simulink model "flux_control_example"  (Simulink 6.3)
settings: Solver=ode3  SolverMode=SingleTasking  StartTime=0.0  StopTime=2  FixedStep=0.02  MaxStep=0.1  MinStep=1e-2  RelTol=1e-2
libraries: simulink x21
settings Model: Creator=JA132999  LastModifiedBy=JA132999  ExtModeAutoUpdateStatusClock=off  BufferReuse=off
settings SolverCC: InitialStep=1e-2
settings MATStruct: SampleTime=0.01  Offset=0  Priority=[1.0]
settings OptimizationCC: BlockReduction=off  BooleanDataType=off  ConditionallyExecuteInputs=off  OptimizeBlockIOStorage=off  BufferReuse=off  ExpressionFolding=off  LocalBlockOutputs=off

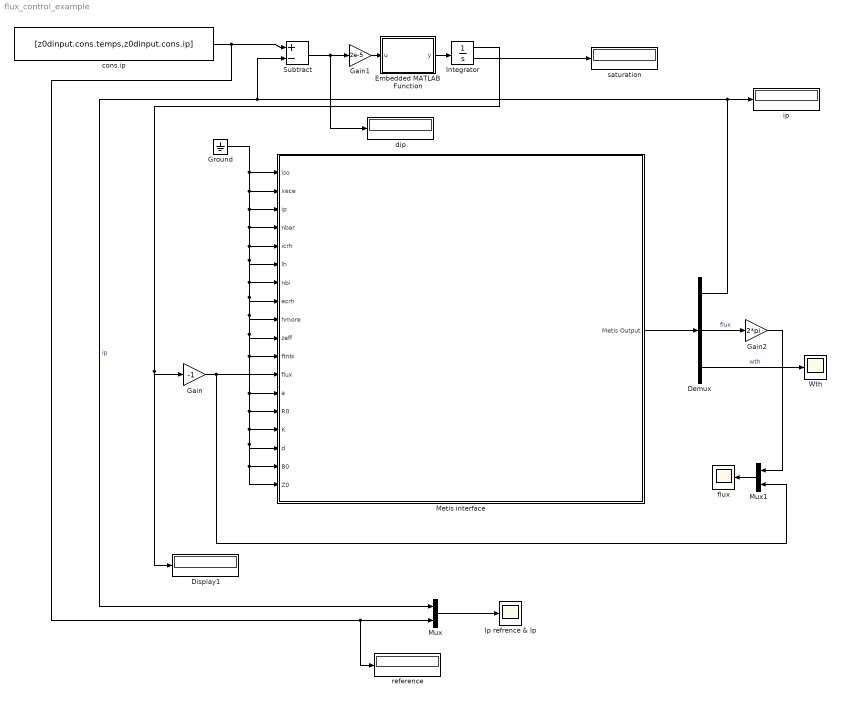
== system flux_control_example ==
  Demux : Demux  Outputs=3
  Display1 : Display
  Embedded MATLAB Function : Stateflow chart
  Gain : Gain  Gain=-1
  Gain1 : Gain  Gain=2e-5
  Gain2 : Gain  Gain=2*pi
  Ground : Ground
  Integrator : Integrator  ShowSaturationPort=on  ZeroCross=off
  Ip refrence & Ip : Scope
      settings: YMin=0  YMax=800000  SaveName=ScopeData3
  Metis interface : Subsystem  AncestorBlock=library_simmetis/Metis interface  TreatAsAtomicUnit=on
  Mux : Mux  Inputs=2
  Mux1 : Mux  Orientation=left  Inputs=2
  Subtract : Sum  Inputs=+-  OutScaling=2^-10
  Wth : Scope
      settings: YMin=0  YMax=100000
  cons.ip : FromWorkspace  VariableName=[z0dinput.cons.temps,z0dinput.cons.ip]  SampleTime=0
  dip : Display
  flux : Scope
      settings: YMin=-2  YMax=0.25
  ip : Display
  reference : Display
  saturation : Display
  wires:
  Ground/1 -> Metis interface/1(iso), Metis interface/2(xece), Metis interface/3(ip), Metis interface/4(nbar), Metis interface/5(icrh), Metis interface/6(lh), Metis interface/7(nbi), Metis interface/8(ecrh), Metis interface/9(hmore), Metis interface/10(zeff), Metis interface/11(ftnbi), Metis interface/13(a), Metis interface/17(B0), Metis interface/14(R0), Metis interface/15(K), Metis interface/18(Z0), Metis interface/16(d)
  Metis interface/1(Metis Output) -> Demux/1
  cons.ip/1 -> Subtract/1, Mux/2, reference/1
  Demux/1 -> Subtract/2, Mux/1, ip/1  "ip"
  Demux/3 -> Wth/1  "wth"
  Demux/2 -> Gain2/1  "flux"
  Integrator/1 -> Gain/1, Display1/1
  Integrator/2 -> saturation/1
  Gain/1 -> Metis interface/12(flux), Mux1/2
  Mux/1 -> Ip refrence & Ip/1
  Subtract/1 -> Gain1/1, dip/1
  Mux1/1 -> flux/1
  Gain2/1 -> Mux1/1
  Gain1/1 -> Embedded MATLAB Function/1(u)
  Embedded MATLAB Function/1(y) -> Integrator/1

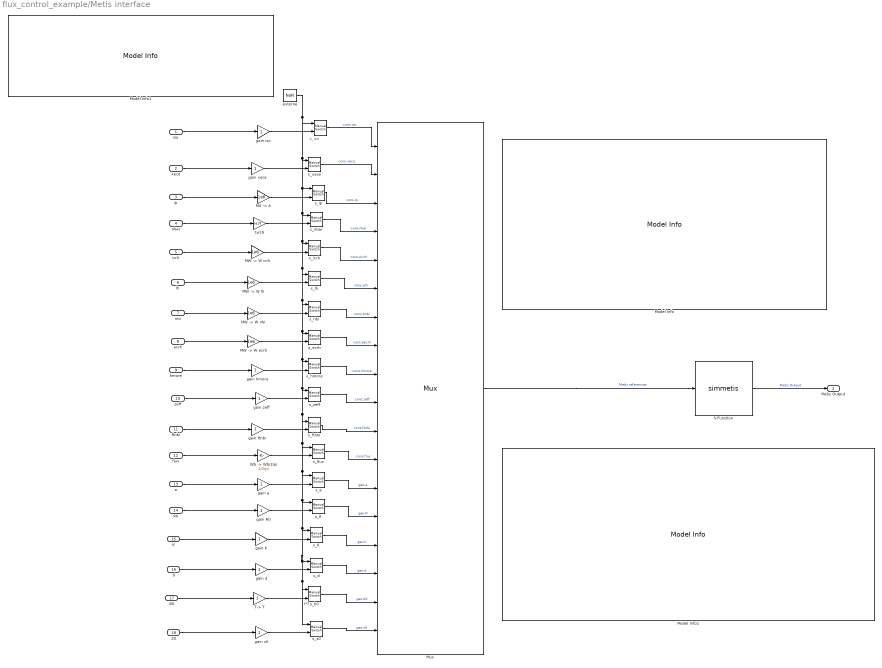
== system flux_control_example/Metis interface ==
  note: s_iso
  iso : Inport
  xece : Inport  Port=2
  ip : Inport  Port=3
  nbar : Inport  Port=4
  icrh : Inport  Port=5
  lh : Inport  Port=6
  nbi : Inport  Port=7
  ecrh : Inport  Port=8
  hmore : Inport  Port=9
  zeff : Inport  Port=10
  ftnbi : Inport  Port=11
  flux : Inport  Port=12
  a : Inport  Port=13
  R0 : Inport  Port=14
  K : Inport  Port=15
  d : Inport  Port=16
  B0 : Inport  Port=17
  Z0 : Inport  Port=18
  " " : simulink/Signal Routing/Manual Switch  sw=1  action=0
  1e19 : Gain  Gain=1e19
  "MA -> A" : Gain  Gain=1e6
  "MW -> W ecrh" : Gain  Gain=1e6
  "MW -> W icrh" : Gain  Gain=1e6
  "MW -> W lh" : Gain  Gain=1e6
  "MW -> W nbi" : Gain  Gain=1e6
  Model Info : simulink/Model-Wide Utilities/Model Info  InitialBlockCM=None  BlockCM=None  Frame=on  DisplayStringWithTags=|  HorizontalTextAlignment=Center  LeftAlignmentValue=0.5  SourceBlockDiagram=flux_control_example  TagMaxNumber=20
      | Interface_SimMetis : Library simmetis interface
      | %<Created>
      | %<ModifiedBy>
      | %<ModifiedDate>
      | %<ModifiedComment>
      | %<Description>
  Model Info1 : simulink/Model-Wide Utilities/Model Info  InitialBlockCM=None  BlockCM=None  Frame=on  DisplayStringWithTags=|  HorizontalTextAlignment=Center  LeftAlignmentValue=0.5  SourceBlockDiagram=flux_control_example  TagMaxNumber=20
      | when an input is set to NaN, 
      | the correspondant reference value
      | is read from Metis file (or data) 
      | and linearely interpolate in time.
  Model Info2 : simulink/Model-Wide Utilities/Model Info  InitialBlockCM=None  BlockCM=None  Frame=on  DisplayStringWithTags=|  HorizontalTextAlignment=Left  LeftAlignmentValue=0.02  SourceBlockDiagram=flux_control_example  TagMaxNumber=20
      | Simmetis parameters :
      | * Metis_file_name : used to parametring Metis in simmetis 
      | (if empty used z0dinput in workspace,
      |  that allow to tune simulation configuration form Metis interface)
      | * list_output : cell array of output names
      | * save_file : results filename (optionnel)
      | * verbose  : if = 1 turn on information writing
  Mux : Mux  Tag=Metis refererences  Inputs=18
      settings: DisplayOption=signals
  S-Function : S-Function  FunctionName=simmetis  Parameters='',{'ip','psi@21','wth'},'',0
  T-> T : Gain
  "Wb -> Wb/2/pi" : Gain  Gain=1/2/pi
  externe : Constant  Value=NaN
  gain K : Gain
  gain R0 : Gain
  gain a : Gain
  gain d : Gain
  gain ftnbi : Gain
  gain hmore : Gain
  gain iso : Gain
  gain xece : Gain
  gain z0 : Gain
  gain zeff : Gain
  s_K : simulink/Signal Routing/Manual Switch  sw=1  action=0
  s_R : simulink/Signal Routing/Manual Switch  sw=1  action=0
  s_a : simulink/Signal Routing/Manual Switch  sw=1  action=0
  s_b0 : simulink/Signal Routing/Manual Switch  sw=1  action=0
  s_d : simulink/Signal Routing/Manual Switch  sw=1  action=0
  s_ecrh : simulink/Signal Routing/Manual Switch  sw=1  action=0
  s_flux : simulink/Signal Routing/Manual Switch  sw=0  action=0
  s_ftnbi : simulink/Signal Routing/Manual Switch  sw=1  action=0
  s_hmore : simulink/Signal Routing/Manual Switch  sw=1  action=0
  s_icrh : simulink/Signal Routing/Manual Switch  sw=1  action=0
  s_ip : simulink/Signal Routing/Manual Switch  sw=1  action=0
  s_lh : simulink/Signal Routing/Manual Switch  sw=1  action=0
  s_nbar : simulink/Signal Routing/Manual Switch  sw=1  action=0
  s_nbi : simulink/Signal Routing/Manual Switch  sw=1  action=0
  s_xece : simulink/Signal Routing/Manual Switch  sw=1  action=0
  s_z0 : simulink/Signal Routing/Manual Switch  sw=1  action=0
  s_zeff : simulink/Signal Routing/Manual Switch  sw=1  action=0
  Metis Output : Outport
  wires:
  s_z0/1 -> Mux/18  "geo.z0"
  s_b0/1 -> Mux/17  "geo.b0"
  gain z0/1 -> s_z0/2
  Z0/1 -> gain z0/1
  s_d/1 -> Mux/16  "geo.d"
  gain d/1 -> s_d/2
  d/1 -> gain d/1
  s_K/1 -> Mux/15  "geo.K"
  gain K/1 -> s_K/2
  K/1 -> gain K/1
  s_R/1 -> Mux/14  "geo.R"
  gain R0/1 -> s_R/2
  R0/1 -> gain R0/1
  s_a/1 -> Mux/13  "geo.a"
  T-> T/1 -> s_b0/2
  B0/1 -> T-> T/1
  gain a/1 -> s_a/2
  a/1 -> gain a/1
  s_flux/1 -> Mux/12  "cons.flux"
  "Wb -> Wb/2/pi"/1 -> s_flux/2
  flux/1 -> "Wb -> Wb/2/pi"/1
  s_ftnbi/1 -> Mux/11  "cons.ftnbi"
  gain ftnbi/1 -> s_ftnbi/2
  ftnbi/1 -> gain ftnbi/1
  s_zeff/1 -> Mux/10  "cons.zeff"
  gain zeff/1 -> s_zeff/2
  zeff/1 -> gain zeff/1
  s_hmore/1 -> Mux/9  "cons.hmore"
  gain hmore/1 -> s_hmore/2
  hmore/1 -> gain hmore/1
  s_ecrh/1 -> Mux/8  "cons.pecrh"
  "MW -> W ecrh"/1 -> s_ecrh/2
  ecrh/1 -> "MW -> W ecrh"/1
  s_nbi/1 -> Mux/7  "cons.pnbi"
  "MW -> W nbi"/1 -> s_nbi/2
  nbi/1 -> "MW -> W nbi"/1
  s_lh/1 -> Mux/6  "cons.plh"
  "MW -> W lh"/1 -> s_lh/2
  lh/1 -> "MW -> W lh"/1
  s_icrh/1 -> Mux/5  "cons.picrh"
  "MW -> W icrh"/1 -> s_icrh/2
  icrh/1 -> "MW -> W icrh"/1
  s_nbar/1 -> Mux/4  "cons.nbar"
  1e19/1 -> s_nbar/2
  nbar/1 -> 1e19/1
  s_ip/1 -> Mux/3  "cons.ip"
  "MA -> A"/1 -> s_ip/2
  ip/1 -> "MA -> A"/1
  gain xece/1 -> s_xece/2
  xece/1 -> gain xece/1
  s_xece/1 -> Mux/2  "cons.xece"
  gain iso/1 -> " "/2
  iso/1 -> gain iso/1
  " "/1 -> Mux/1  "cons.iso"
  externe/1 -> s_z0/1, s_b0/1, s_d/1, s_K/1, s_R/1, s_a/1, s_flux/1, s_ftnbi/1, s_zeff/1, s_hmore/1, s_ecrh/1, s_nbi/1, s_lh/1, s_icrh/1, s_nbar/1, s_ip/1, s_xece/1, " "/1  "ext"
  Mux/1 -> S-Function/1  "Metis references"
  S-Function/1 -> Metis Output/1  "Metis Output"

== matlab function Embedded MATLAB Function ==
  data: u input inherited; y output inherited
function y = fcn(u)
% This block supports an embeddable subset of the MATLAB language.
% See the help menu for details. 

y = max(-20,min(20,u));
